simulink model "w2prob3"  (R2020a)
settings: Solver=VariableStepAuto  StartTime=0.0  StopTime=120  RelTol=1e-3
PostLoadFcn:
  | m = 1000;
  | b = 50;
  | u = 500;
settings Model: DataDictionary=w2prob3vars.sldd  Creator=Anjali123  LastModifiedBy=Anjali123

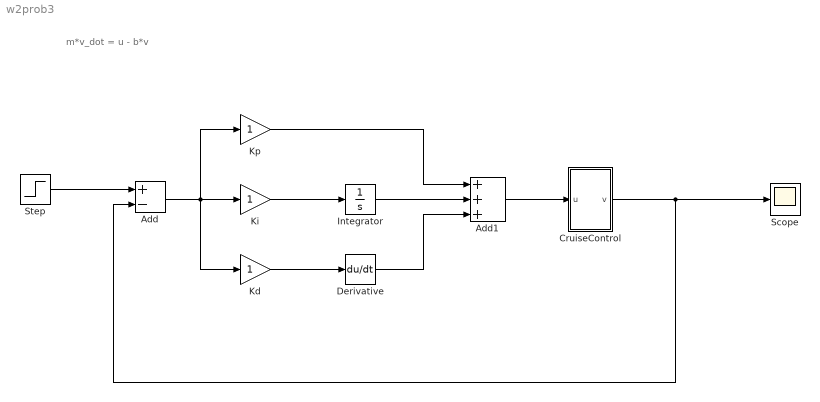
== system w2prob3 ==
  note: m*v_dot = u - b*v
  Add : Sum  Inputs=+-
  Add1 : Sum  Inputs=+++
  CruiseControl : Subsystem
  Derivative : Derivative
  Integrator : Integrator
  Kd : Gain
  Ki : Gain
  Kp : Gain
  "Scope " : Scope
  "Step " : Step  Time=0  After=u  SampleTime=0
  wires:
  CruiseControl/1(v) -> Add/2, "Scope "/1
  "Step "/1 -> Add/1
  Add1/1 -> CruiseControl/1(u)
  Add/1 -> Kp/1, Kd/1, Ki/1
  Ki/1 -> Integrator/1
  Integrator/1 -> Add1/2
  Kd/1 -> Derivative/1
  Derivative/1 -> Add1/3
  Kp/1 -> Add1/1

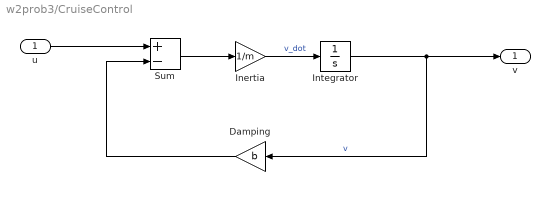
== system w2prob3/CruiseControl ==
  u : Inport
  Damping : Gain  Gain=b
  Inertia : Gain  Gain=1/m
  "Integrator " : Integrator
  "Sum " : Sum  Inputs=+-
  v : Outport
  wires:
  Inertia/1 -> "Integrator "/1  "v_dot"
  "Sum "/1 -> Inertia/1
  "Integrator "/1 -> v/1, Damping/1  "v"
  u/1 -> "Sum "/1
  Damping/1 -> "Sum "/2
